simulink model "ex3"  (R2024a)
settings: Solver=FixedStepAuto  StartTime=0.0  StopTime=15.0  FixedStep=1e-5  RelTol=1e-5
undefined symbols (not defined in the file or in its folder): A, B, Bf, C, Cz, D, Dz, G, K1, K2, Lw, Lx, w_0, x_0
settings Model: Creator=admin  LastModifiedBy=anton
settings RTWCC: GPUComputeCapability=3.5

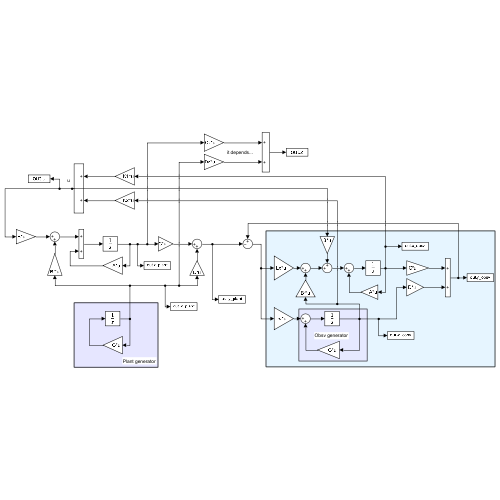
[thumbnail: Simulink's stored preview of the top-level diagram]
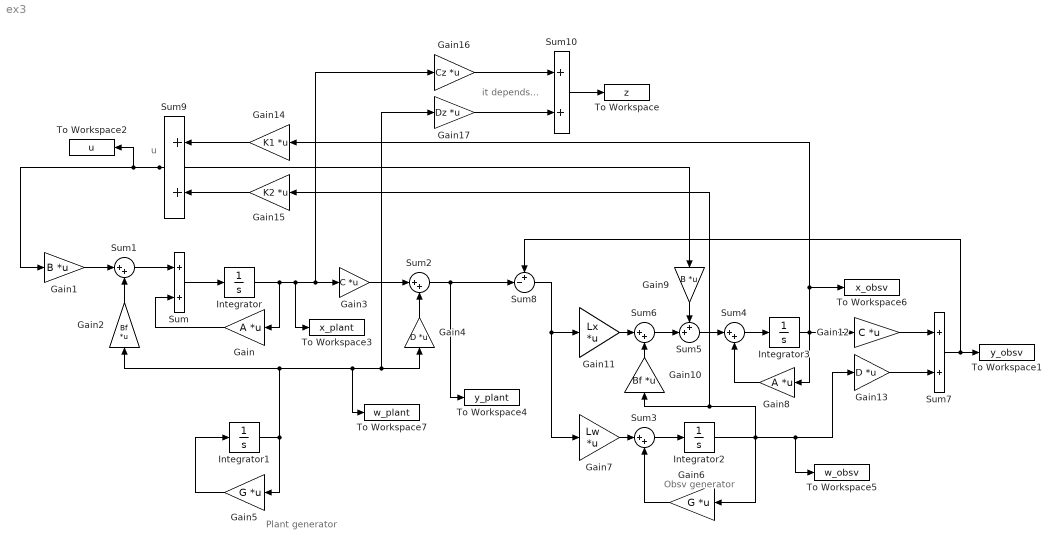
== system ex3 ==
  note: it depends...
  note: Obsv generator
  note: u
  note: Plant generator
  Gain : Gain  Gain=A  Multiplication=Matrix(K*u)
  Gain1 : Gain  Gain=B  Multiplication=Matrix(K*u)
  Gain10 : Gain  Gain=Bf  Multiplication=Matrix(K*u)
  Gain11 : Gain  Gain=Lx  Multiplication=Matrix(K*u)
  Gain12 : Gain  Gain=C  Multiplication=Matrix(K*u)
  Gain13 : Gain  Gain=D  Multiplication=Matrix(K*u)
  Gain14 : Gain  Gain=K1  Multiplication=Matrix(K*u)
  Gain15 : Gain  Gain=K2  Multiplication=Matrix(K*u)
  Gain16 : Gain  Gain=Cz  Multiplication=Matrix(K*u)
  Gain17 : Gain  Gain=Dz  Multiplication=Matrix(K*u)
  Gain2 : Gain  Gain=Bf  Multiplication=Matrix(K*u)
  Gain3 : Gain  Gain=C  Multiplication=Matrix(K*u)
  Gain4 : Gain  Gain=D  Multiplication=Matrix(K*u)
  Gain5 : Gain  Gain=G  Multiplication=Matrix(K*u)
  Gain6 : Gain  Gain=G  Multiplication=Matrix(K*u)
  Gain7 : Gain  Gain=Lw  Multiplication=Matrix(K*u)
  Gain8 : Gain  Gain=A  Multiplication=Matrix(K*u)
  Gain9 : Gain  Gain=B  Multiplication=Matrix(K*u)
  Integrator : Integrator  InitialCondition=x_0
  Integrator1 : Integrator  InitialCondition=w_0
  Integrator2 : Integrator
  Integrator3 : Integrator
  Sum{,7,9..10} (4 alike) : Sum
  Sum{1..4,6} (5 alike) : Sum  Inputs=|++
  Sum5 : Sum  Inputs=++|
  Sum8 : Sum  Inputs=+-|
  To Workspace : ToWorkspace  VariableName=z  SaveFormat=Timeseries  SampleTime=-1
  To Workspace1 : ToWorkspace  VariableName=y_obsv  SaveFormat=Timeseries  SampleTime=-1
  To Workspace2 : ToWorkspace  VariableName=u  SaveFormat=Timeseries  SampleTime=-1
  To Workspace3 : ToWorkspace  VariableName=x_plant  SaveFormat=Timeseries  SampleTime=-1
  To Workspace4 : ToWorkspace  VariableName=y_plant  SaveFormat=Timeseries  SampleTime=-1
  To Workspace5 : ToWorkspace  VariableName=w_obsv  SaveFormat=Timeseries  SampleTime=-1
  To Workspace6 : ToWorkspace  VariableName=x_obsv  SaveFormat=Timeseries  SampleTime=-1
  To Workspace7 : ToWorkspace  VariableName=w_plant  SaveFormat=Timeseries  SampleTime=-1
  wires:
  Sum/1 -> Integrator/1
  Gain/1 -> Sum/2
  Integrator/1 -> To Workspace3/1, Gain16/1, Gain3/1, Gain/1
  Sum1/1 -> Sum/1
  Gain1/1 -> Sum1/1
  Gain2/1 -> Sum1/2
  Gain3/1 -> Sum2/1
  Gain4/1 -> Sum2/2
  Integrator1/1 -> Gain2/1, To Workspace7/1, Gain17/1, Gain4/1, Gain5/1
  Gain5/1 -> Integrator1/1
  Integrator2/1 -> Gain15/1, Gain10/1, To Workspace5/1, Gain13/1, Gain6/1
  Sum3/1 -> Integrator2/1
  Gain6/1 -> Sum3/2
  Gain7/1 -> Sum3/1
  Sum4/1 -> Integrator3/1
  Gain8/1 -> Sum4/2
  Integrator3/1 -> To Workspace6/1, Gain14/1, Gain12/1, Gain8/1
  Sum5/1 -> Sum4/1
  Gain10/1 -> Sum6/2
  Gain11/1 -> Sum6/1
  Sum6/1 -> Sum5/2
  Gain9/1 -> Sum5/1
  Gain13/1 -> Sum7/2
  Gain12/1 -> Sum7/1
  Sum2/1 -> To Workspace4/1, Sum8/2
  Sum7/1 -> To Workspace1/1, Sum8/1
  Sum8/1 -> Gain11/1, Gain7/1
  Gain14/1 -> Sum9/1
  Gain15/1 -> Sum9/2
  Sum9/1 -> To Workspace2/1, Gain1/1, Gain9/1
  Gain17/1 -> Sum10/2
  Gain16/1 -> Sum10/1
  Sum10/1 -> To Workspace/1
